simulink model "ssc_battery_management_R2020a"  (R2020a)
settings: Solver=daessc  StartTime=0.0  StopTime=2000  FixedStep=0.1  MinStep=1e-6  RelTol=1e-5  EnableMultiTasking=on
PreLoadFcn:
  | ModelPath = fileparts(get_param(bdroot,'FileName'));
  | addpath(ModelPath);
  | 
  | ssc_battery_management_R2012b_ini
values from neighbouring files (symbols this model uses):
  AltData100AMaxCurrent =     [AlternatorTableData.mat]
  AltData100AVoltage =     [AlternatorTableData.mat]
  AltData80AMaxCurrent =     [AlternatorTableData.mat]
  AltData80AVoltage =     [AlternatorTableData.mat]
  Kt = [0.80,1.10,1.20,1.12;]    [ssc_lead_acid_battery_50Ah_ini.m]    (also in ssc_lead_acid_battery_80Ah_ini.m)
  Kt_Temps = [25 40 60 75]    [ssc_lead_acid_battery_50Ah_ini.m]    (also in ssc_lead_acid_battery_80Ah_ini.m)
  theta_f = -40    [ssc_lead_acid_battery_50Ah_ini.m]    (also in ssc_lead_acid_battery_80Ah_ini.m)
  theta_init = 25    [ssc_lead_acid_battery_50Ah_ini.m]    (also in ssc_lead_acid_battery_80Ah_ini.m)
undefined symbols (not defined in the file or in its folder): beta, center, DiscIntNeverNeededParam, exponent, polyTerms, sigbuilder_block, WendlandNumTerms, width
libraries: fl_lib x130, LeadAcidBattery_lib x36, nesl_utility x28, simulink x6
(part 3 of 4)

== system ssc_battery_management_R2020a/Lead-Acid Battery/Battery Cell 5/Thermal Model ==
  Battery thermal mass : fl_lib/Thermal/Thermal Elements/Thermal Mass  mass=1 kg  sp_heat=Ctheta J/kg/K  T_specify=on  T_priority=High  T=theta_init+273 K  T_nominal_specify=off  T_nominal_unit=K  T_nominal_value=1  Q_specify=off  Q_priority=None  Q=0 W  Q_nominal_specify=off  Q_nominal_unit=W  Q_nominal_value=1
  Ideal Temperature Sensor : fl_lib/Thermal/Thermal Sensors/Temperature Sensor
  Ideal Heat Flow Source : fl_lib/Thermal/Thermal Sources/Controlled Heat Flow Rate Source
  Kt as a function of temperature : fl_lib/Physical Signals/Lookup Tables/PS Lookup Table (1D)  x=[theta_f, Kt_Temps]+273 K  f=[0 Kt]  interp_method=simscape.enum.interpolation.linear  extrap_method=simscape.enum.extrapolation.nearest
      settings: SourceProductBaseCode=SS
  Thermal Reference1 : fl_lib/Thermal/Thermal Elements/Thermal Reference
  Thermal Reference2 : fl_lib/Thermal/Thermal Elements/Thermal Reference
  Ps : PMIOPort  Tag=PMCPort  Side=Left
  H : PMIOPort  Tag=PMCPort  Port=2  Side=Left
  Kt : PMIOPort  Tag=PMCPort  Port=3  Side=Right
  T : PMIOPort  Tag=PMCPort  Port=4  Side=Right
  connections:
  Ideal Temperature Sensor/RConn1 -- Thermal Reference2/LConn1
  Ideal Temperature Sensor/RConn2 -- Kt as a function of temperature/LConn1 -- T/RConn1
  Thermal Reference1/LConn1 -- Ideal Heat Flow Source/RConn2
  H/RConn1 -- Ideal Temperature Sensor/LConn1 -- Ideal Heat Flow Source/LConn1 -- Battery thermal mass/LConn1
  Kt/RConn1 -- Kt as a function of temperature/RConn1
  Ideal Heat Flow Source/RConn1 -- Ps/RConn1

== system ssc_battery_management_R2020a/Lead-Acid Battery/Battery Cell 6/Thermal Model ==
  Battery thermal mass : fl_lib/Thermal/Thermal Elements/Thermal Mass  mass=1 kg  sp_heat=Ctheta J/kg/K  T_specify=on  T_priority=High  T=theta_init+273 K  T_nominal_specify=off  T_nominal_unit=K  T_nominal_value=1  Q_specify=off  Q_priority=None  Q=0 W  Q_nominal_specify=off  Q_nominal_unit=W  Q_nominal_value=1
  Ideal Temperature Sensor : fl_lib/Thermal/Thermal Sensors/Temperature Sensor
  Ideal Heat Flow Source : fl_lib/Thermal/Thermal Sources/Controlled Heat Flow Rate Source
  Kt as a function of temperature : fl_lib/Physical Signals/Lookup Tables/PS Lookup Table (1D)  x=[theta_f, Kt_Temps]+273 K  f=[0 Kt]  interp_method=simscape.enum.interpolation.linear  extrap_method=simscape.enum.extrapolation.nearest
      settings: SourceProductBaseCode=SS
  Thermal Reference1 : fl_lib/Thermal/Thermal Elements/Thermal Reference
  Thermal Reference2 : fl_lib/Thermal/Thermal Elements/Thermal Reference
  Ps : PMIOPort  Tag=PMCPort  Side=Left
  H : PMIOPort  Tag=PMCPort  Port=2  Side=Left
  Kt : PMIOPort  Tag=PMCPort  Port=3  Side=Right
  T : PMIOPort  Tag=PMCPort  Port=4  Side=Right
  connections:
  Ideal Temperature Sensor/RConn1 -- Thermal Reference2/LConn1
  Ideal Temperature Sensor/RConn2 -- Kt as a function of temperature/LConn1 -- T/RConn1
  Thermal Reference1/LConn1 -- Ideal Heat Flow Source/RConn2
  H/RConn1 -- Ideal Temperature Sensor/LConn1 -- Ideal Heat Flow Source/LConn1 -- Battery thermal mass/LConn1
  Kt/RConn1 -- Kt as a function of temperature/RConn1
  Ideal Heat Flow Source/RConn1 -- Ps/RConn1

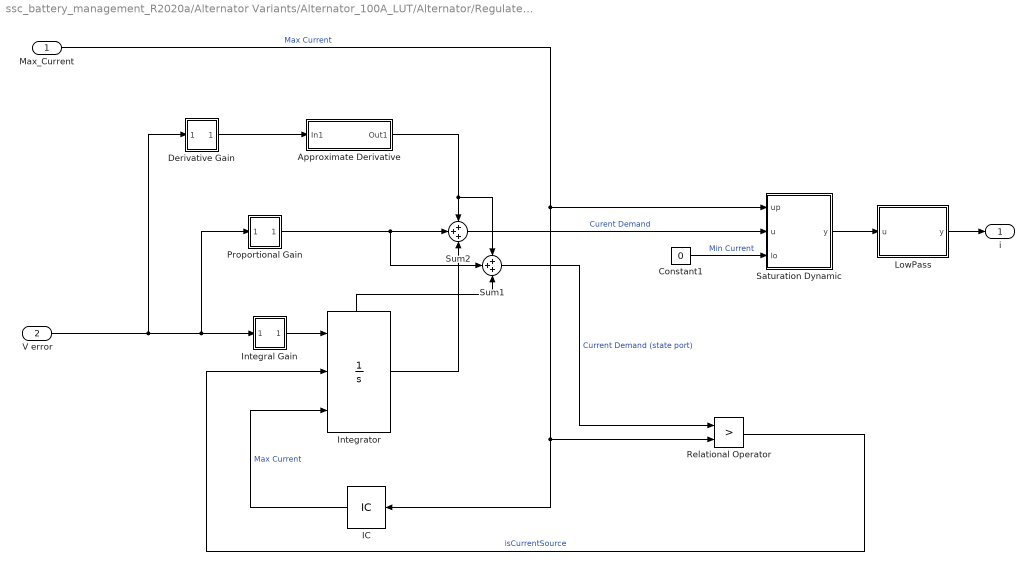
== system ssc_battery_management_R2020a/Alternator Variants/Alternator_100A_LUT/Alternator/Regulate Voltage ==
  Max_Current : Inport
  V error : Inport  Port=2
  Approximate Derivative : Subsystem
  Constant1 : Constant  Value=0  OutDataTypeStr=double
  Derivative Gain : Subsystem  LoadFcn=slideg Load  mask(Slider Gain){low=0, gain=22, high=200}
      settings: CopyFcn=slideg Copy  DeleteFcn=slideg DeleteBlock  NameChangeFcn=slideg NameChange  OpenFcn=slideg Open  CloseFcn=slideg Close  ParentCloseFcn=slideg ParentClose
      mask Display: disp(gain)
  IC : InitialCondition  Value=i_init
  Integral Gain : Subsystem  LoadFcn=slideg Load  mask(Slider Gain){low=0, gain=40, high=200}
      settings: CopyFcn=slideg Copy  DeleteFcn=slideg DeleteBlock  NameChangeFcn=slideg NameChange  OpenFcn=slideg Open  CloseFcn=slideg Close  ParentCloseFcn=slideg ParentClose
      mask Display: disp(gain)
  Integrator : Integrator  ExternalReset=falling  InitialConditionSource=external  LimitOutput=on  UpperSaturationLimit=140  LowerSaturationLimit=0  ShowStatePort=on  IgnoreLimit=on
  LowPass : Subsystem  mask{T=0.3, IC=i_init}
      mask prompts: T "Time Constant"; IC "Initial Condition"
      mask Display:
      | disp(...
      |     strvcat(['1/(' num2str(T) 's+1)'],...
      | ['IC=' num2str(IC)])...
      | )
  Proportional Gain : Subsystem  LoadFcn=slideg Load  mask(Slider Gain){low=0, gain=40, high=200}
      settings: CopyFcn=slideg Copy  DeleteFcn=slideg DeleteBlock  NameChangeFcn=slideg NameChange  OpenFcn=slideg Open  CloseFcn=slideg Close  ParentCloseFcn=slideg ParentClose
      mask Display: disp(gain)
  Relational Operator : RelationalOperator  Operator=>  OutDataTypeStr=boolean  RndMeth=Nearest
  Saturation Dynamic : Subsystem  mask(Saturation Dynamic){}
      mask help: Bound the range of the second input by using the first input (upper limit) and the third input (lower limit).
      mask Display: plot([0.15 0.85],[.5 .5],[.5 .5],[0.05 0.95],0.15+0.7*[0 .25 .75 1],0.05+0.9*[.25 .25 .75 .75]);
  Sum1 : Sum  Inputs=+++
  Sum2 : Sum  Inputs=+++
  i : Outport
  wires:
  Sum2/1 -> Saturation Dynamic/2(u)  "Curent Demand"
  Proportional Gain/1(Out1) -> Sum2/2, Sum1/2
  Integral Gain/1(Out1) -> Integrator/1
  Integrator/1 -> Sum2/3
  V error/1 -> Integral Gain/1(In1), Proportional Gain/1(In1), Derivative Gain/1(In1)
  Max_Current/1 -> Saturation Dynamic/1(up), Relational Operator/2, IC/1  "Max Current"
  Constant1/1 -> Saturation Dynamic/3(lo)  "Min Current"
  Saturation Dynamic/1(y) -> LowPass/1(u)
  Relational Operator/1 -> Integrator/2  "isCurrentSource"
  IC/1 -> Integrator/3  "Max Current"
  Approximate Derivative/1(Out1) -> Sum2/1, Sum1/1
  Derivative Gain/1(Out1) -> Approximate Derivative/1(In1)
  Integrator/State -> Sum1/3
  Sum1/1 -> Relational Operator/1  "Current Demand (state port)"
  LowPass/1(y) -> i/1

== system ssc_battery_management_R2020a/Alternator Variants/Alternator_100A_MBC/Alternator/100A_Max_Current ==
  Temp : Inport
  Voltage : Inport  Port=2
  RPM : Inport  Port=3
  Constraint Block : Subsystem
  Mx1 : Mux  Inputs=3
  xregrbf : Subsystem
      mask init:
      | xregmaskinitialization;
  Max_Current : Outport
  Constraints : Outport  Port=2
  wires:
  Constraint Block/1(C) -> Constraints/1
  xregrbf/1(Y) -> Max_Current/1
  Mx1/1 -> Constraint Block/1(X), xregrbf/1(X)
  RPM/1 -> Mx1/3
  Voltage/1 -> Mx1/2
  Temp/1 -> Mx1/1

== system ssc_battery_management_R2020a/Alternator Variants/Alternator_100A_MBC/Alternator/100A_Voltage ==
  Temp : Inport
  Load : Inport  Port=2
  RPM : Inport  Port=3
  Constraint Block : Subsystem
  Mx1 : Mux  Inputs=3
  xregrbf : Subsystem
      mask init:
      | xregmaskinitialization;
  Voltage : Outport
  Constraints : Outport  Port=2
  wires:
  Constraint Block/1(C) -> Constraints/1
  xregrbf/1(Y) -> Voltage/1
  Mx1/1 -> Constraint Block/1(X), xregrbf/1(X)
  RPM/1 -> Mx1/3
  Load/1 -> Mx1/2
  Temp/1 -> Mx1/1

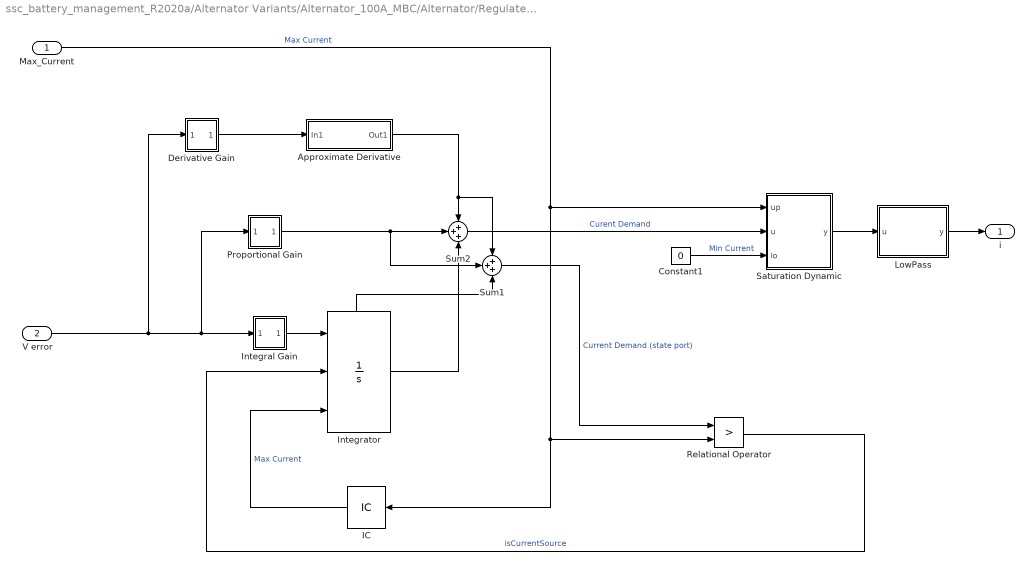
== system ssc_battery_management_R2020a/Alternator Variants/Alternator_100A_MBC/Alternator/Regulate Voltage ==
  Max_Current : Inport
  V error : Inport  Port=2
  Approximate Derivative : Subsystem
  Constant1 : Constant  Value=0  OutDataTypeStr=double
  Derivative Gain : Subsystem  LoadFcn=slideg Load  mask(Slider Gain){low=0, gain=22, high=200}
      settings: CopyFcn=slideg Copy  DeleteFcn=slideg DeleteBlock  NameChangeFcn=slideg NameChange  OpenFcn=slideg Open  CloseFcn=slideg Close  ParentCloseFcn=slideg ParentClose
      mask Display: disp(gain)
  IC : InitialCondition  Value=i_init
  Integral Gain : Subsystem  LoadFcn=slideg Load  mask(Slider Gain){low=0, gain=40, high=200}
      settings: CopyFcn=slideg Copy  DeleteFcn=slideg DeleteBlock  NameChangeFcn=slideg NameChange  OpenFcn=slideg Open  CloseFcn=slideg Close  ParentCloseFcn=slideg ParentClose
      mask Display: disp(gain)
  Integrator : Integrator  ExternalReset=falling  InitialConditionSource=external  LimitOutput=on  UpperSaturationLimit=140  LowerSaturationLimit=0  ShowStatePort=on  IgnoreLimit=on
  LowPass : Subsystem  mask{T=0.3, IC=i_init}
      mask prompts: T "Time Constant"; IC "Initial Condition"
      mask Display:
      | disp(...
      |     strvcat(['1/(' num2str(T) 's+1)'],...
      | ['IC=' num2str(IC)])...
      | )
  Proportional Gain : Subsystem  LoadFcn=slideg Load  mask(Slider Gain){low=0, gain=40, high=200}
      settings: CopyFcn=slideg Copy  DeleteFcn=slideg DeleteBlock  NameChangeFcn=slideg NameChange  OpenFcn=slideg Open  CloseFcn=slideg Close  ParentCloseFcn=slideg ParentClose
      mask Display: disp(gain)
  Relational Operator : RelationalOperator  Operator=>  OutDataTypeStr=boolean  RndMeth=Nearest
  Saturation Dynamic : Subsystem  mask(Saturation Dynamic){}
      mask help: Bound the range of the second input by using the first input (upper limit) and the third input (lower limit).
      mask Display: plot([0.15 0.85],[.5 .5],[.5 .5],[0.05 0.95],0.15+0.7*[0 .25 .75 1],0.05+0.9*[.25 .25 .75 .75]);
  Sum1 : Sum  Inputs=+++
  Sum2 : Sum  Inputs=+++
  i : Outport
  wires:
  LowPass/1(y) -> i/1
  Sum1/1 -> Relational Operator/1  "Current Demand (state port)"
  Integrator/State -> Sum1/3
  Derivative Gain/1(Out1) -> Approximate Derivative/1(In1)
  Approximate Derivative/1(Out1) -> Sum1/1, Sum2/1
  IC/1 -> Integrator/3  "Max Current"
  Relational Operator/1 -> Integrator/2  "isCurrentSource"
  Saturation Dynamic/1(y) -> LowPass/1(u)
  Constant1/1 -> Saturation Dynamic/3(lo)  "Min Current"
  Max_Current/1 -> IC/1, Relational Operator/2, Saturation Dynamic/1(up)  "Max Current"
  V error/1 -> Derivative Gain/1(In1), Proportional Gain/1(In1), Integral Gain/1(In1)
  Integrator/1 -> Sum2/3
  Integral Gain/1(Out1) -> Integrator/1
  Proportional Gain/1(Out1) -> Sum1/2, Sum2/2
  Sum2/1 -> Saturation Dynamic/2(u)  "Curent Demand"

== system ssc_battery_management_R2020a/Alternator Variants/Alternator_80A_LUT/Alternator/Regulate Voltage ==
  Max_Current : Inport
  V error : Inport  Port=2
  Approximate Derivative : Subsystem
  Constant1 : Constant  Value=0  OutDataTypeStr=double
  Derivative Gain : simulink/Math Operations/Slider Gain  gain=1  low=0  high=200
  IC : InitialCondition  Value=i_init
  Integral Gain : simulink/Math Operations/Slider Gain  gain=1  low=0  high=200
  Integrator : Integrator  ExternalReset=falling  InitialConditionSource=external  LimitOutput=on  UpperSaturationLimit=140  LowerSaturationLimit=0  ShowStatePort=on  IgnoreLimit=on
  LowPass : Subsystem  mask{T=0.3, IC=i_init}
      mask prompts: T "Time Constant"; IC "Initial Condition"
      mask Display:
      | disp(...
      |     strvcat(['1/(' num2str(T) 's+1)'],...
      | ['IC=' num2str(IC)])...
      | )
  Proportional Gain : simulink/Math Operations/Slider Gain  gain=1  low=0  high=200
  Relational Operator : RelationalOperator  Operator=>  OutDataTypeStr=boolean  RndMeth=Nearest
  Saturation Dynamic : simulink/Discontinuities/Saturation Dynamic  OutMin=[]  OutMax=[]  OutDataTypeStr=Inherit: Same as second input  OutDataType=fixdt(1, 16)  OutScaling=2^-10  DoSatur=off
  Sum1 : Sum  Inputs=+++
  Sum2 : Sum  Inputs=+++
  i : Outport
  wires:
  LowPass/1(y) -> i/1
  Sum1/1 -> Relational Operator/1  "Current Demand (state port)"
  Integrator/State -> Sum1/3
  Derivative Gain/1 -> Approximate Derivative/1(In1)
  Approximate Derivative/1(Out1) -> Sum1/1, Sum2/1
  IC/1 -> Integrator/3  "Max Current"
  Relational Operator/1 -> Integrator/2  "isCurrentSource"
  Saturation Dynamic/1 -> LowPass/1(u)
  Constant1/1 -> Saturation Dynamic/3  "Min Current"
  Max_Current/1 -> IC/1, Relational Operator/2, Saturation Dynamic/1  "Max Current"
  V error/1 -> Derivative Gain/1, Proportional Gain/1, Integral Gain/1
  Integrator/1 -> Sum2/3
  Integral Gain/1 -> Integrator/1
  Proportional Gain/1 -> Sum1/2, Sum2/2
  Sum2/1 -> Saturation Dynamic/2  "Curent Demand"

== system ssc_battery_management_R2020a/Alternator Variants/Alternator_80A_MBC/Alternator/80A_Max_Current ==
  Temp : Inport
  Voltage : Inport  Port=2
  RPM : Inport  Port=3
  Constraint Block : Subsystem
  Mx1 : Mux  Inputs=3
  xregrbf : Subsystem
      mask init:
      | xregmaskinitialization;
  Max_Current : Outport
  Constraints : Outport  Port=2
  wires:
  Constraint Block/1(C) -> Constraints/1
  xregrbf/1(Y) -> Max_Current/1
  Mx1/1 -> Constraint Block/1(X), xregrbf/1(X)
  RPM/1 -> Mx1/3
  Voltage/1 -> Mx1/2
  Temp/1 -> Mx1/1

== system ssc_battery_management_R2020a/Alternator Variants/Alternator_80A_MBC/Alternator/80A_Voltage ==
  Temp : Inport
  Load : Inport  Port=2
  RPM : Inport  Port=3
  Constraint Block : Subsystem
  Mx1 : Mux  Inputs=3
  xregrbf : Subsystem
      mask init:
      | xregmaskinitialization;
  Voltage : Outport
  Constraints : Outport  Port=2
  wires:
  Constraint Block/1(C) -> Constraints/1
  xregrbf/1(Y) -> Voltage/1
  Mx1/1 -> Constraint Block/1(X), xregrbf/1(X)
  RPM/1 -> Mx1/3
  Load/1 -> Mx1/2
  Temp/1 -> Mx1/1

== system ssc_battery_management_R2020a/Alternator Variants/Alternator_80A_MBC/Alternator/Regulate Voltage ==
  Max_Current : Inport
  V error : Inport  Port=2
  Approximate Derivative : Subsystem
  Constant1 : Constant  Value=0  OutDataTypeStr=double
  Derivative Gain : Subsystem  LoadFcn=slideg Load  mask(Slider Gain){low=0, gain=22, high=200}
      settings: CopyFcn=slideg Copy  DeleteFcn=slideg DeleteBlock  NameChangeFcn=slideg NameChange  OpenFcn=slideg Open  CloseFcn=slideg Close  ParentCloseFcn=slideg ParentClose
      mask Display: disp(gain)
  IC : InitialCondition  Value=i_init
  Integral Gain : Subsystem  LoadFcn=slideg Load  mask(Slider Gain){low=0, gain=40, high=200}
      settings: CopyFcn=slideg Copy  DeleteFcn=slideg DeleteBlock  NameChangeFcn=slideg NameChange  OpenFcn=slideg Open  CloseFcn=slideg Close  ParentCloseFcn=slideg ParentClose
      mask Display: disp(gain)
  Integrator : Integrator  ExternalReset=falling  InitialConditionSource=external  LimitOutput=on  UpperSaturationLimit=140  LowerSaturationLimit=0  ShowStatePort=on  IgnoreLimit=on
  LowPass : Subsystem  mask{T=0.3, IC=i_init}
      mask prompts: T "Time Constant"; IC "Initial Condition"
      mask Display:
      | disp(...
      |     strvcat(['1/(' num2str(T) 's+1)'],...
      | ['IC=' num2str(IC)])...
      | )
  Proportional Gain : Subsystem  LoadFcn=slideg Load  mask(Slider Gain){low=0, gain=40, high=200}
      settings: CopyFcn=slideg Copy  DeleteFcn=slideg DeleteBlock  NameChangeFcn=slideg NameChange  OpenFcn=slideg Open  CloseFcn=slideg Close  ParentCloseFcn=slideg ParentClose
      mask Display: disp(gain)
  Relational Operator : RelationalOperator  Operator=>  OutDataTypeStr=boolean  RndMeth=Nearest
  Saturation Dynamic : Subsystem  mask(Saturation Dynamic){}
      mask help: Bound the range of the second input by using the first input (upper limit) and the third input (lower limit).
      mask Display: plot([0.15 0.85],[.5 .5],[.5 .5],[0.05 0.95],0.15+0.7*[0 .25 .75 1],0.05+0.9*[.25 .25 .75 .75]);
  Sum1 : Sum  Inputs=+++
  Sum2 : Sum  Inputs=+++
  i : Outport
  wires:
  Sum2/1 -> Saturation Dynamic/2(u)  "Curent Demand"
  Proportional Gain/1(Out1) -> Sum2/2, Sum1/2
  Integral Gain/1(Out1) -> Integrator/1
  Integrator/1 -> Sum2/3
  V error/1 -> Integral Gain/1(In1), Proportional Gain/1(In1), Derivative Gain/1(In1)
  Max_Current/1 -> Saturation Dynamic/1(up), Relational Operator/2, IC/1  "Max Current"
  Constant1/1 -> Saturation Dynamic/3(lo)  "Min Current"
  Saturation Dynamic/1(y) -> LowPass/1(u)
  Relational Operator/1 -> Integrator/2  "isCurrentSource"
  IC/1 -> Integrator/3  "Max Current"
  Approximate Derivative/1(Out1) -> Sum2/1, Sum1/1
  Derivative Gain/1(Out1) -> Approximate Derivative/1(In1)
  Integrator/State -> Sum1/3
  Sum1/1 -> Relational Operator/1  "Current Demand (state port)"
  LowPass/1(y) -> i/1

== system ssc_battery_management_R2020a/Alternator Variants/Alternator_100A_LUT/Alternator/Regulate Voltage/Approximate Derivative ==
  In1 : Inport
  Derivative Gain : Subsystem  LoadFcn=slideg Load  mask(Slider Gain){low=0, gain=38, high=200}
      settings: CopyFcn=slideg Copy  DeleteFcn=slideg DeleteBlock  NameChangeFcn=slideg NameChange  OpenFcn=slideg Open  CloseFcn=slideg Close  ParentCloseFcn=slideg ParentClose
      mask Display: disp(gain)
  Filter : Integrator
  Sum3 : Sum  Inputs=|+-  InputSameDT=on  SaturateOnIntegerOverflow=on  OutDataTypeStr=Inherit: Same as first input
  Out1 : Outport
  wires:
  In1/1 -> Sum3/1
  Filter/1 -> Sum3/2
  Derivative Gain/1(Out1) -> Out1/1, Filter/1
  Sum3/1 -> Derivative Gain/1(In1)

== system ssc_battery_management_R2020a/Alternator Variants/Alternator_100A_LUT/Alternator/Regulate Voltage/Derivative Gain ==
  In1 : Inport
  Slider Gain : Gain  Gain=gain  SaturateOnIntegerOverflow=on  OutDataTypeStr=Inherit: Same as input  ParamDataTypeStr=Inherit: Same as input
  Out1 : Outport
  wires:
  In1/1 -> Slider Gain/1
  Slider Gain/1 -> Out1/1

== system ssc_battery_management_R2020a/Alternator Variants/Alternator_100A_LUT/Alternator/Regulate Voltage/Integral Gain ==
  In1 : Inport
  Slider Gain : Gain  Gain=gain  SaturateOnIntegerOverflow=on  OutDataTypeStr=Inherit: Same as input  ParamDataTypeStr=Inherit: Same as input
  Out1 : Outport
  wires:
  Slider Gain/1 -> Out1/1
  In1/1 -> Slider Gain/1

== system ssc_battery_management_R2020a/Alternator Variants/Alternator_100A_LUT/Alternator/Regulate Voltage/LowPass ==
  u : Inport
  Gain : Gain  Gain=1/T
  Integrator : Integrator  InitialCondition=IC
  Sum : Sum  Inputs=|+-
  y : Outport
  wires:
  Gain/1 -> Integrator/1  "ydot"
  u/1 -> Sum/1
  Sum/1 -> Gain/1  "ydot"
  Integrator/1 -> y/1, Sum/2  "y"

== system ssc_battery_management_R2020a/Alternator Variants/Alternator_100A_LUT/Alternator/Regulate Voltage/Proportional Gain ==
  In1 : Inport
  Slider Gain : Gain  Gain=gain  SaturateOnIntegerOverflow=on  OutDataTypeStr=Inherit: Same as input  ParamDataTypeStr=Inherit: Same as input
  Out1 : Outport
  wires:
  Slider Gain/1 -> Out1/1
  In1/1 -> Slider Gain/1

== system ssc_battery_management_R2020a/Alternator Variants/Alternator_100A_LUT/Alternator/Regulate Voltage/Saturation Dynamic ==
  up : Inport
  u : Inport  Port=2
  lo : Inport  Port=3
  Enforce lower limit : MinMax  Function=max  Inputs=2  OutDataTypeStr=Inherit: Inherit via back propagation  ZeroCross=off
  Enforce upper limit : MinMax  Inputs=2  OutDataTypeStr=Inherit: Inherit via back propagation  ZeroCross=off
  FixPt Data Type Duplicate : S-Function  FunctionName=sfix_dtprop  Parameters=15,NumInputPorts  SFunctionDeploymentMode=off  EnableBusSupport=off  mask(Data Type Duplicate){NumInputPorts=3}
      mask prompts: NumInputPorts "Number of input ports:"
      mask help: Force all inputs to have the exact same data type.
      mask Display: fprintf('Same\nDT')
  y : Outport
  wires:
  lo/1 -> Enforce lower limit/1
  Enforce lower limit/1 -> FixPt Data Type Duplicate/2, Enforce upper limit/1
  u/1 -> Enforce lower limit/2, FixPt Data Type Duplicate/3
  up/1 -> Enforce upper limit/2
  Enforce upper limit/1 -> y/1, FixPt Data Type Duplicate/1

== system ssc_battery_management_R2020a/Alternator Variants/Alternator_100A_MBC/Alternator/100A_Max_Current/Constraint Block ==
  X : Inport
  Constraints : Subsystem
  Term : Terminator
  C : Outport
  wires:
  Constraints/2(Distances) -> C/1
  Constraints/1(Status) -> Term/1
  X/1 -> Constraints/1(Factors)

== system ssc_battery_management_R2020a/Alternator Variants/Alternator_100A_MBC/Alternator/100A_Max_Current/xregrbf ==
  X : Inport
  Code : Subsystem
  Saturation : Saturate  UpperLimit=1  LowerLimit=-1  ZeroCross=off
  rbfwendlandEval : Subsystem  mask{NumTerms=WendlandNumTerms, E=exponent, P=polyTerms, B=beta, S=width, C=center}
      mask prompts: NumTerms "Number of Poylnomial Terms"; E "Exponent"; P "Polynomial Terms"; B "Betas"; S "Widths"; C "Centers"
  term : Terminator
  Y : Outport
  wires:
  Saturation/1 -> rbfwendlandEval/1(X)
  rbfwendlandEval/2(J) -> term/1
  rbfwendlandEval/1(Y) -> Y/1
  Code/1(XCoded) -> Saturation/1
  X/1 -> Code/1(XIn)

== system ssc_battery_management_R2020a/Alternator Variants/Alternator_100A_MBC/Alternator/100A_Voltage/Constraint Block ==
  X : Inport
  Constraints : Subsystem
  Term : Terminator
  C : Outport
  wires:
  Constraints/2(Distances) -> C/1
  Constraints/1(Status) -> Term/1
  X/1 -> Constraints/1(Factors)

== system ssc_battery_management_R2020a/Alternator Variants/Alternator_100A_MBC/Alternator/100A_Voltage/xregrbf ==
  X : Inport
  Code : Subsystem
  Saturation : Saturate  UpperLimit=1  LowerLimit=-1  ZeroCross=off
  rbfwendlandEval : Subsystem  mask{NumTerms=WendlandNumTerms, E=exponent, P=polyTerms, B=beta, S=width, C=center}
      mask prompts: NumTerms "Number of Poylnomial Terms"; E "Exponent"; P "Polynomial Terms"; B "Betas"; S "Widths"; C "Centers"
  term : Terminator
  Y : Outport
  wires:
  Saturation/1 -> rbfwendlandEval/1(X)
  rbfwendlandEval/2(J) -> term/1
  rbfwendlandEval/1(Y) -> Y/1
  Code/1(XCoded) -> Saturation/1
  X/1 -> Code/1(XIn)

== system ssc_battery_management_R2020a/Alternator Variants/Alternator_100A_MBC/Alternator/Regulate Voltage/Approximate Derivative ==
  In1 : Inport
  Derivative Gain : Subsystem  LoadFcn=slideg Load  mask(Slider Gain){low=0, gain=38, high=200}
      settings: CopyFcn=slideg Copy  DeleteFcn=slideg DeleteBlock  NameChangeFcn=slideg NameChange  OpenFcn=slideg Open  CloseFcn=slideg Close  ParentCloseFcn=slideg ParentClose
      mask Display: disp(gain)
  Filter : Integrator
  Sum3 : Sum  Inputs=|+-  InputSameDT=on  SaturateOnIntegerOverflow=on  OutDataTypeStr=Inherit: Same as first input
  Out1 : Outport
  wires:
  Sum3/1 -> Derivative Gain/1(In1)
  Derivative Gain/1(Out1) -> Filter/1, Out1/1
  Filter/1 -> Sum3/2
  In1/1 -> Sum3/1

== system ssc_battery_management_R2020a/Alternator Variants/Alternator_100A_MBC/Alternator/Regulate Voltage/Derivative Gain ==
  In1 : Inport
  Slider Gain : Gain  Gain=gain  SaturateOnIntegerOverflow=on  OutDataTypeStr=Inherit: Same as input  ParamDataTypeStr=Inherit: Same as input
  Out1 : Outport
  wires:
  Slider Gain/1 -> Out1/1
  In1/1 -> Slider Gain/1

== system ssc_battery_management_R2020a/Alternator Variants/Alternator_100A_MBC/Alternator/Regulate Voltage/Integral Gain ==
  In1 : Inport
  Slider Gain : Gain  Gain=gain  SaturateOnIntegerOverflow=on  OutDataTypeStr=Inherit: Same as input  ParamDataTypeStr=Inherit: Same as input
  Out1 : Outport
  wires:
  In1/1 -> Slider Gain/1
  Slider Gain/1 -> Out1/1

== system ssc_battery_management_R2020a/Alternator Variants/Alternator_100A_MBC/Alternator/Regulate Voltage/LowPass ==
  u : Inport
  Gain : Gain  Gain=1/T
  Integrator : Integrator  InitialCondition=IC
  Sum : Sum  Inputs=|+-
  y : Outport
  wires:
  Integrator/1 -> Sum/2, y/1  "y"
  Sum/1 -> Gain/1  "ydot"
  u/1 -> Sum/1
  Gain/1 -> Integrator/1  "ydot"

== system ssc_battery_management_R2020a/Alternator Variants/Alternator_100A_MBC/Alternator/Regulate Voltage/Proportional Gain ==
  In1 : Inport
  Slider Gain : Gain  Gain=gain  SaturateOnIntegerOverflow=on  OutDataTypeStr=Inherit: Same as input  ParamDataTypeStr=Inherit: Same as input
  Out1 : Outport
  wires:
  In1/1 -> Slider Gain/1
  Slider Gain/1 -> Out1/1

== system ssc_battery_management_R2020a/Alternator Variants/Alternator_100A_MBC/Alternator/Regulate Voltage/Saturation Dynamic ==
  up : Inport
  u : Inport  Port=2
  lo : Inport  Port=3
  Enforce lower limit : MinMax  Function=max  Inputs=2  OutDataTypeStr=Inherit: Inherit via back propagation  ZeroCross=off
  Enforce upper limit : MinMax  Inputs=2  OutDataTypeStr=Inherit: Inherit via back propagation  ZeroCross=off
  FixPt Data Type Duplicate : S-Function  FunctionName=sfix_dtprop  Parameters=15,NumInputPorts  SFunctionDeploymentMode=off  EnableBusSupport=off  mask(Data Type Duplicate){NumInputPorts=3}
      mask prompts: NumInputPorts "Number of input ports:"
      mask help: Force all inputs to have the exact same data type.
      mask Display: fprintf('Same\nDT')
  y : Outport
  wires:
  Enforce upper limit/1 -> FixPt Data Type Duplicate/1, y/1
  up/1 -> Enforce upper limit/2
  u/1 -> FixPt Data Type Duplicate/3, Enforce lower limit/2
  Enforce lower limit/1 -> Enforce upper limit/1, FixPt Data Type Duplicate/2
  lo/1 -> Enforce lower limit/1

== system ssc_battery_management_R2020a/Alternator Variants/Alternator_80A_LUT/Alternator/Regulate Voltage/Approximate Derivative ==
  In1 : Inport
  Derivative Gain : simulink/Math Operations/Slider Gain  gain=1  low=0  high=200
  Filter : Integrator
  Sum3 : Sum  Inputs=|+-  InputSameDT=on  SaturateOnIntegerOverflow=on  OutDataTypeStr=Inherit: Same as first input
  Out1 : Outport
  wires:
  Sum3/1 -> Derivative Gain/1
  Derivative Gain/1 -> Filter/1, Out1/1
  Filter/1 -> Sum3/2
  In1/1 -> Sum3/1

== system ssc_battery_management_R2020a/Alternator Variants/Alternator_80A_LUT/Alternator/Regulate Voltage/LowPass ==
  u : Inport
  Gain : Gain  Gain=1/T
  Integrator : Integrator  InitialCondition=IC
  Sum : Sum  Inputs=|+-
  y : Outport
  wires:
  Integrator/1 -> Sum/2, y/1  "y"
  Sum/1 -> Gain/1  "ydot"
  u/1 -> Sum/1
  Gain/1 -> Integrator/1  "ydot"

== system ssc_battery_management_R2020a/Alternator Variants/Alternator_80A_MBC/Alternator/80A_Max_Current/Constraint Block ==
  X : Inport
  Constraints : Subsystem
  Term : Terminator
  C : Outport
  wires:
  Constraints/2(Distances) -> C/1
  Constraints/1(Status) -> Term/1
  X/1 -> Constraints/1(Factors)

== system ssc_battery_management_R2020a/Alternator Variants/Alternator_80A_MBC/Alternator/80A_Max_Current/xregrbf ==
  X : Inport
  Code : Subsystem
  Saturation : Saturate  UpperLimit=1  LowerLimit=-1  ZeroCross=off
  rbflogisticrbfEval : Subsystem  mask{B=beta, S=width, C=center}
      mask prompts: B "Betas"; S "Widths"; C "Centers"
  term : Terminator
  Y : Outport
  wires:
  Saturation/1 -> rbflogisticrbfEval/1(X)
  rbflogisticrbfEval/2(J) -> term/1
  rbflogisticrbfEval/1(Y) -> Y/1
  Code/1(XCoded) -> Saturation/1
  X/1 -> Code/1(XIn)

== system ssc_battery_management_R2020a/Alternator Variants/Alternator_80A_MBC/Alternator/80A_Voltage/Constraint Block ==
  X : Inport
  Constraints : Subsystem
  Term : Terminator
  C : Outport
  wires:
  Constraints/2(Distances) -> C/1
  Constraints/1(Status) -> Term/1
  X/1 -> Constraints/1(Factors)

== system ssc_battery_management_R2020a/Alternator Variants/Alternator_80A_MBC/Alternator/80A_Voltage/xregrbf ==
  X : Inport
  Code : Subsystem
  Saturation : Saturate  UpperLimit=1  LowerLimit=-1  ZeroCross=off
  rbfwendlandEval : Subsystem  mask{NumTerms=WendlandNumTerms, E=exponent, P=polyTerms, B=beta, S=width, C=center}
      mask prompts: NumTerms "Number of Poylnomial Terms"; E "Exponent"; P "Polynomial Terms"; B "Betas"; S "Widths"; C "Centers"
  term : Terminator
  Y : Outport
  wires:
  Saturation/1 -> rbfwendlandEval/1(X)
  rbfwendlandEval/2(J) -> term/1
  rbfwendlandEval/1(Y) -> Y/1
  Code/1(XCoded) -> Saturation/1
  X/1 -> Code/1(XIn)

== system ssc_battery_management_R2020a/Alternator Variants/Alternator_80A_MBC/Alternator/Regulate Voltage/Approximate Derivative ==
  In1 : Inport
  Derivative Gain : Subsystem  LoadFcn=slideg Load  mask(Slider Gain){low=0, gain=38, high=200}
      settings: CopyFcn=slideg Copy  DeleteFcn=slideg DeleteBlock  NameChangeFcn=slideg NameChange  OpenFcn=slideg Open  CloseFcn=slideg Close  ParentCloseFcn=slideg ParentClose
      mask Display: disp(gain)
  Filter : Integrator
  Sum3 : Sum  Inputs=|+-  InputSameDT=on  SaturateOnIntegerOverflow=on  OutDataTypeStr=Inherit: Same as first input
  Out1 : Outport
  wires:
  In1/1 -> Sum3/1
  Filter/1 -> Sum3/2
  Derivative Gain/1(Out1) -> Out1/1, Filter/1
  Sum3/1 -> Derivative Gain/1(In1)

== system ssc_battery_management_R2020a/Alternator Variants/Alternator_80A_MBC/Alternator/Regulate Voltage/Derivative Gain ==
  In1 : Inport
  Slider Gain : Gain  Gain=gain  SaturateOnIntegerOverflow=on  OutDataTypeStr=Inherit: Same as input  ParamDataTypeStr=Inherit: Same as input
  Out1 : Outport
  wires:
  In1/1 -> Slider Gain/1
  Slider Gain/1 -> Out1/1

== system ssc_battery_management_R2020a/Alternator Variants/Alternator_80A_MBC/Alternator/Regulate Voltage/Integral Gain ==
  In1 : Inport
  Slider Gain : Gain  Gain=gain  SaturateOnIntegerOverflow=on  OutDataTypeStr=Inherit: Same as input  ParamDataTypeStr=Inherit: Same as input
  Out1 : Outport
  wires:
  Slider Gain/1 -> Out1/1
  In1/1 -> Slider Gain/1

== system ssc_battery_management_R2020a/Alternator Variants/Alternator_80A_MBC/Alternator/Regulate Voltage/LowPass ==
  u : Inport
  Gain : Gain  Gain=1/T
  Integrator : Integrator  InitialCondition=IC
  Sum : Sum  Inputs=|+-
  y : Outport
  wires:
  Gain/1 -> Integrator/1  "ydot"
  u/1 -> Sum/1
  Sum/1 -> Gain/1  "ydot"
  Integrator/1 -> y/1, Sum/2  "y"

== system ssc_battery_management_R2020a/Alternator Variants/Alternator_80A_MBC/Alternator/Regulate Voltage/Proportional Gain ==
  In1 : Inport
  Slider Gain : Gain  Gain=gain  SaturateOnIntegerOverflow=on  OutDataTypeStr=Inherit: Same as input  ParamDataTypeStr=Inherit: Same as input
  Out1 : Outport
  wires:
  Slider Gain/1 -> Out1/1
  In1/1 -> Slider Gain/1

== system ssc_battery_management_R2020a/Alternator Variants/Alternator_80A_MBC/Alternator/Regulate Voltage/Saturation Dynamic ==
  up : Inport
  u : Inport  Port=2
  lo : Inport  Port=3
  Enforce lower limit : MinMax  Function=max  Inputs=2  OutDataTypeStr=Inherit: Inherit via back propagation  ZeroCross=off
  Enforce upper limit : MinMax  Inputs=2  OutDataTypeStr=Inherit: Inherit via back propagation  ZeroCross=off
  FixPt Data Type Duplicate : S-Function  FunctionName=sfix_dtprop  Parameters=15,NumInputPorts  SFunctionDeploymentMode=off  EnableBusSupport=off  mask(Data Type Duplicate){NumInputPorts=3}
      mask prompts: NumInputPorts "Number of input ports:"
      mask help: Force all inputs to have the exact same data type.
      mask Display: fprintf('Same\nDT')
  y : Outport
  wires:
  lo/1 -> Enforce lower limit/1
  Enforce lower limit/1 -> FixPt Data Type Duplicate/2, Enforce upper limit/1
  u/1 -> Enforce lower limit/2, FixPt Data Type Duplicate/3
  up/1 -> Enforce upper limit/2
  Enforce upper limit/1 -> y/1, FixPt Data Type Duplicate/1

== system ssc_battery_management_R2020a/Alternator Variants/Alternator_100A_LUT/Alternator/Regulate Voltage/Approximate Derivative/Derivative Gain ==
  In1 : Inport
  Slider Gain : Gain  Gain=gain  SaturateOnIntegerOverflow=on  OutDataTypeStr=Inherit: Same as input  ParamDataTypeStr=Inherit: Same as input
  Out1 : Outport
  wires:
  In1/1 -> Slider Gain/1
  Slider Gain/1 -> Out1/1

== system ssc_battery_management_R2020a/Alternator Variants/Alternator_100A_MBC/Alternator/100A_Max_Current/Constraint Block/Constraints ==
  Factors : Inport
  Compare : RelationalOperator  Operator=<=  RndMeth=Nearest  InputSameDT=on
  Constant : Constant  Value=0
  Constraint : Subsystem  mask(MBC Constraint){}
      mask help: This is a constraint generated by the Model-Based Calibration Toolbox.
      mask Display:
      | disp( 'MBC\nConstraint' )
      | port_label( 'output', 1, 'In/Out' )
  T : Terminator
  Status : Outport
  Distances : Outport  Port=2
  wires:
  Constraint/2(Interior Point) -> T/1
  Constraint/1(Distance) -> Compare/1, Distances/1
  Factors/1 -> Constraint/1(Xin)
  Compare/1 -> Status/1
  Constant/1 -> Compare/2

== system ssc_battery_management_R2020a/Alternator Variants/Alternator_100A_MBC/Alternator/100A_Max_Current/xregrbf/Code ==
  XIn : Inport
  Mid : Constant  Value=[45 12.75 3500 ]
  demux : Demux  Outputs=3
      settings: DisplayOption=none
  gain : Gain  Gain=[0.0153846153846154 0.8 0.0004 ]  SaturateOnIntegerOverflow=on  OutDataTypeStr=Inherit: Same as input  ParamDataTypeStr=Inherit: Same as input
  mux : Mux  Inputs=3
  sum : Sum  Inputs=-+|  InputSameDT=on  SaturateOnIntegerOverflow=on  OutDataTypeStr=Inherit: Same as first input
  XCoded : Outport
  wires:
  gain/1 -> XCoded/1
  sum/1 -> gain/1
  mux/1 -> sum/2
  XIn/1 -> demux/1
  Mid/1 -> sum/1
  demux/3 -> mux/3
  demux/2 -> mux/2
  demux/1 -> mux/1

== system ssc_battery_management_R2020a/Alternator Variants/Alternator_100A_MBC/Alternator/100A_Max_Current/xregrbf/rbfwendlandEval ==
  X : Inport
  Constant13 : Constant  Value=P
  Constant14 : Constant  Value=E
  Constant2 : Constant  Value=S  VectorParams1D=off
  Constant3 : Constant  Value=B
  Constant4 : Constant  Value=C  VectorParams1D=off
  Math Function4 : Math  Operator=sqrt  SignedPower=on  SaturateOnIntegerOverflow=on
  Product4 : Product  Multiplication=Matrix(*)  InputSameDT=on  SaturateOnIntegerOverflow=on  OutDataTypeStr=Inherit: Same as first input
  R : Subsystem
  Wendland : Subsystem  mask{NumTerms=NumTerms}
      mask prompts: NumTerms "Number of Polynomial Terms"
  Y : Outport
  J : Outport  Port=2
  wires:
  Constant14/1 -> Wendland/3(Exponent)
  Product4/1 -> Y/1
  Wendland/1(P) -> J/1, Product4/1
  Constant3/1 -> Product4/2
  Math Function4/1 -> Wendland/1(R/S)
  Constant4/1 -> R/2("Centers ")
  X/1 -> R/1(X)
  Constant2/1 -> R/3(S)
  R/1((R/S)^2) -> Math Function4/1
  Constant13/1 -> Wendland/2(PolyTerms)

== system ssc_battery_management_R2020a/Alternator Variants/Alternator_100A_MBC/Alternator/100A_Voltage/Constraint Block/Constraints ==
  Factors : Inport
  Compare : RelationalOperator  Operator=<=  RndMeth=Nearest  InputSameDT=on
  Constant : Constant  Value=0
  Constraint : Subsystem  mask(MBC Constraint){}
      mask help: This is a constraint generated by the Model-Based Calibration Toolbox.
      mask Display:
      | disp( 'MBC\nConstraint' )
      | port_label( 'output', 1, 'In/Out' )
  T : Terminator
  Status : Outport
  Distances : Outport  Port=2
  wires:
  Constraint/2(Interior Point) -> T/1
  Constraint/1(Distance) -> Compare/1, Distances/1
  Factors/1 -> Constraint/1(Xin)
  Compare/1 -> Status/1
  Constant/1 -> Compare/2

== system ssc_battery_management_R2020a/Alternator Variants/Alternator_100A_MBC/Alternator/100A_Voltage/xregrbf/Code ==
  XIn : Inport
  Mid : Constant  Value=[45 70 3500 ]
  demux : Demux  Outputs=3
      settings: DisplayOption=none
  gain : Gain  Gain=[0.0153846153846154 0.02 0.0004 ]  SaturateOnIntegerOverflow=on  OutDataTypeStr=Inherit: Same as input  ParamDataTypeStr=Inherit: Same as input
  mux : Mux  Inputs=3
  sum : Sum  Inputs=-+|  InputSameDT=on  SaturateOnIntegerOverflow=on  OutDataTypeStr=Inherit: Same as first input
  XCoded : Outport
  wires:
  gain/1 -> XCoded/1
  sum/1 -> gain/1
  mux/1 -> sum/2
  XIn/1 -> demux/1
  Mid/1 -> sum/1
  demux/3 -> mux/3
  demux/2 -> mux/2
  demux/1 -> mux/1

== system ssc_battery_management_R2020a/Alternator Variants/Alternator_100A_MBC/Alternator/100A_Voltage/xregrbf/rbfwendlandEval ==
  X : Inport
  Constant13 : Constant  Value=P
  Constant14 : Constant  Value=E
  Constant2 : Constant  Value=S  VectorParams1D=off
  Constant3 : Constant  Value=B
  Constant4 : Constant  Value=C  VectorParams1D=off
  Math Function4 : Math  Operator=sqrt  SignedPower=on  SaturateOnIntegerOverflow=on
  Product4 : Product  Multiplication=Matrix(*)  InputSameDT=on  SaturateOnIntegerOverflow=on  OutDataTypeStr=Inherit: Same as first input
  R : Subsystem
  Wendland : Subsystem  mask{NumTerms=NumTerms}
      mask prompts: NumTerms "Number of Polynomial Terms"
  Y : Outport
  J : Outport  Port=2
  wires:
  Constant14/1 -> Wendland/3(Exponent)
  Product4/1 -> Y/1
  Wendland/1(P) -> J/1, Product4/1
  Constant3/1 -> Product4/2
  Math Function4/1 -> Wendland/1(R/S)
  Constant4/1 -> R/2("Centers ")
  X/1 -> R/1(X)
  Constant2/1 -> R/3(S)
  R/1((R/S)^2) -> Math Function4/1
  Constant13/1 -> Wendland/2(PolyTerms)

== system ssc_battery_management_R2020a/Alternator Variants/Alternator_100A_MBC/Alternator/Regulate Voltage/Approximate Derivative/Derivative Gain ==
  In1 : Inport
  Slider Gain : Gain  Gain=gain  SaturateOnIntegerOverflow=on  OutDataTypeStr=Inherit: Same as input  ParamDataTypeStr=Inherit: Same as input
  Out1 : Outport
  wires:
  Slider Gain/1 -> Out1/1
  In1/1 -> Slider Gain/1

== system ssc_battery_management_R2020a/Alternator Variants/Alternator_80A_MBC/Alternator/80A_Max_Current/Constraint Block/Constraints ==
  Factors : Inport
  Compare : RelationalOperator  Operator=<=  RndMeth=Nearest  InputSameDT=on
  Constant : Constant  Value=0
  Constraint : Subsystem  mask(MBC Constraint){}
      mask help: This is a constraint generated by the Model-Based Calibration Toolbox.
      mask Display:
      | disp( 'MBC\nConstraint' )
      | port_label( 'output', 1, 'In/Out' )
  T : Terminator
  Status : Outport
  Distances : Outport  Port=2
  wires:
  Constraint/2(Interior Point) -> T/1
  Constraint/1(Distance) -> Compare/1, Distances/1
  Factors/1 -> Constraint/1(Xin)
  Compare/1 -> Status/1
  Constant/1 -> Compare/2

== system ssc_battery_management_R2020a/Alternator Variants/Alternator_80A_MBC/Alternator/80A_Max_Current/xregrbf/Code ==
  XIn : Inport
  Mid : Constant  Value=[35 12.75 3500 ]
  demux : Demux  Outputs=3
      settings: DisplayOption=none
  gain : Gain  Gain=[0.0181818181818182 0.8 0.0004 ]  SaturateOnIntegerOverflow=on  OutDataTypeStr=Inherit: Same as input  ParamDataTypeStr=Inherit: Same as input
  mux : Mux  Inputs=3
  sum : Sum  Inputs=-+|  InputSameDT=on  SaturateOnIntegerOverflow=on  OutDataTypeStr=Inherit: Same as first input
  XCoded : Outport
  wires:
  gain/1 -> XCoded/1
  sum/1 -> gain/1
  mux/1 -> sum/2
  XIn/1 -> demux/1
  Mid/1 -> sum/1
  demux/3 -> mux/3
  demux/2 -> mux/2
  demux/1 -> mux/1

== system ssc_battery_management_R2020a/Alternator Variants/Alternator_80A_MBC/Alternator/80A_Max_Current/xregrbf/rbflogisticrbfEval ==
  X : Inport
  Constant2 : Constant  Value=S  VectorParams1D=off
  Constant3 : Constant  Value=B
  Constant4 : Constant  Value=C  VectorParams1D=off
  Logistic : Subsystem
  Math Function4 : Math  Operator=sqrt  SignedPower=on  SaturateOnIntegerOverflow=on
  Product4 : Product  Multiplication=Matrix(*)  InputSameDT=on  SaturateOnIntegerOverflow=on  OutDataTypeStr=Inherit: Same as first input
  R : Subsystem
  Y : Outport
  J : Outport  Port=2
  wires:
  Math Function4/1 -> Logistic/1(R/S)
  Constant3/1 -> Product4/2
  R/1((R/S)^2) -> Math Function4/1
  Logistic/1(P) -> J/1, Product4/1
  Product4/1 -> Y/1
  Constant4/1 -> R/2("Centers ")
  X/1 -> R/1(X)
  Constant2/1 -> R/3(S)

== system ssc_battery_management_R2020a/Alternator Variants/Alternator_80A_MBC/Alternator/80A_Voltage/Constraint Block/Constraints ==
  Factors : Inport
  Compare : RelationalOperator  Operator=<=  RndMeth=Nearest  InputSameDT=on
  Constant : Constant  Value=0
  Constraint : Subsystem  mask(MBC Constraint){}
      mask help: This is a constraint generated by the Model-Based Calibration Toolbox.
      mask Display:
      | disp( 'MBC\nConstraint' )
      | port_label( 'output', 1, 'In/Out' )
  T : Terminator
  Status : Outport
  Distances : Outport  Port=2
  wires:
  Constraint/2(Interior Point) -> T/1
  Constraint/1(Distance) -> Compare/1, Distances/1
  Factors/1 -> Constraint/1(Xin)
  Compare/1 -> Status/1
  Constant/1 -> Compare/2

== system ssc_battery_management_R2020a/Alternator Variants/Alternator_80A_MBC/Alternator/80A_Voltage/xregrbf/Code ==
  XIn : Inport
  Mid : Constant  Value=[45 70 3500 ]
  demux : Demux  Outputs=3
      settings: DisplayOption=none
  gain : Gain  Gain=[0.0153846153846154 0.02 0.0004 ]  SaturateOnIntegerOverflow=on  OutDataTypeStr=Inherit: Same as input  ParamDataTypeStr=Inherit: Same as input
  mux : Mux  Inputs=3
  sum : Sum  Inputs=-+|  InputSameDT=on  SaturateOnIntegerOverflow=on  OutDataTypeStr=Inherit: Same as first input
  XCoded : Outport
  wires:
  gain/1 -> XCoded/1
  sum/1 -> gain/1
  mux/1 -> sum/2
  XIn/1 -> demux/1
  Mid/1 -> sum/1
  demux/3 -> mux/3
  demux/2 -> mux/2
  demux/1 -> mux/1

== system ssc_battery_management_R2020a/Alternator Variants/Alternator_80A_MBC/Alternator/80A_Voltage/xregrbf/rbfwendlandEval ==
  X : Inport
  Constant13 : Constant  Value=P
  Constant14 : Constant  Value=E
  Constant2 : Constant  Value=S  VectorParams1D=off
  Constant3 : Constant  Value=B
  Constant4 : Constant  Value=C  VectorParams1D=off
  Math Function4 : Math  Operator=sqrt  SignedPower=on  SaturateOnIntegerOverflow=on
  Product4 : Product  Multiplication=Matrix(*)  InputSameDT=on  SaturateOnIntegerOverflow=on  OutDataTypeStr=Inherit: Same as first input
  R : Subsystem
  Wendland : Subsystem  mask{NumTerms=NumTerms}
      mask prompts: NumTerms "Number of Polynomial Terms"
  Y : Outport
  J : Outport  Port=2
  wires:
  Constant14/1 -> Wendland/3(Exponent)
  Product4/1 -> Y/1
  Wendland/1(P) -> J/1, Product4/1
  Constant3/1 -> Product4/2
  Math Function4/1 -> Wendland/1(R/S)
  Constant4/1 -> R/2("Centers ")
  X/1 -> R/1(X)
  Constant2/1 -> R/3(S)
  R/1((R/S)^2) -> Math Function4/1
  Constant13/1 -> Wendland/2(PolyTerms)

== system ssc_battery_management_R2020a/Alternator Variants/Alternator_80A_MBC/Alternator/Regulate Voltage/Approximate Derivative/Derivative Gain ==
  In1 : Inport
  Slider Gain : Gain  Gain=gain  SaturateOnIntegerOverflow=on  OutDataTypeStr=Inherit: Same as input  ParamDataTypeStr=Inherit: Same as input
  Out1 : Outport
  wires:
  In1/1 -> Slider Gain/1
  Slider Gain/1 -> Out1/1

== system ssc_battery_management_R2020a/Alternator Variants/Alternator_100A_MBC/Alternator/100A_Max_Current/Constraint Block/Constraints/Constraint ==
  Xin : Inport
  Constraint - conrange : Subsystem  mask(Range Constraint){}
      mask help: This block impements range constraints for MBC models
      mask init:
      | ud = get_param( gcb, 'UserData' );M = ud.M;HW = ud.HW;LB = ud.LB;UB = ud.UB;Scale = ud.Scale;
  switch : Switch  SaturateOnIntegerOverflow=on  InputSameDT=on
  Distance : Outport
  Interior Point : Outport  Port=2
  wires:
  Constraint - conrange/2(Interior Point) -> switch/1
  Constraint - conrange/1(Distance) -> switch/2, Distance/1
  Xin/1 -> Constraint - conrange/1(Xin), switch/3
  switch/1 -> Interior Point/1

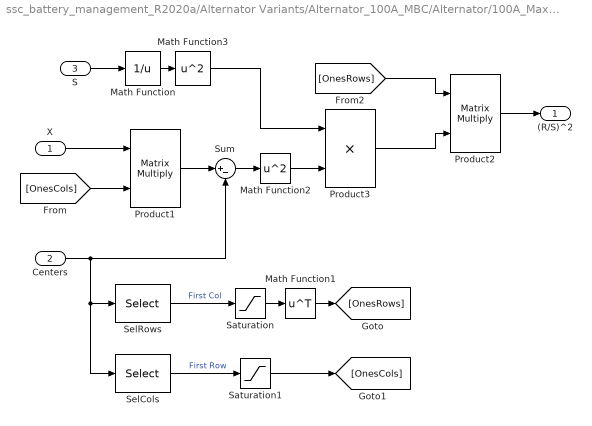
== system ssc_battery_management_R2020a/Alternator Variants/Alternator_100A_MBC/Alternator/100A_Max_Current/xregrbf/rbfwendlandEval/R ==
  X : Inport
  "Centers " : Inport  Port=2
  S : Inport  Port=3
  Math Function : Math  Operator=reciprocal  SignedPower=on  SaturateOnIntegerOverflow=on
  Math Function1 : Math  Operator=transpose  SignedPower=on  SaturateOnIntegerOverflow=on
  Math Function2 : Math  Operator=square  SignedPower=on  SaturateOnIntegerOverflow=on
  Math Function3 : Math  Operator=square  SignedPower=on  SaturateOnIntegerOverflow=on
  Product1 : Product  Multiplication=Matrix(*)  InputSameDT=on  SaturateOnIntegerOverflow=on  OutDataTypeStr=Inherit: Same as first input
  Product2 : Product  Multiplication=Matrix(*)  InputSameDT=on  SaturateOnIntegerOverflow=on  OutDataTypeStr=Inherit: Same as first input
  Product3 : Product  InputSameDT=on  SaturateOnIntegerOverflow=on  OutDataTypeStr=Inherit: Same as first input
  Saturation : Saturate  UpperLimit=1  LowerLimit=1
  Saturation1 : Saturate  UpperLimit=1  LowerLimit=1
  SelCols : Selector  NumberOfDimensions=2  InputPortWidth=3  IndexOptions=Index vector (dialog),Select all  Indices=1,-1  OutputSizes=1
  SelRows : Selector  NumberOfDimensions=2  InputPortWidth=3  IndexOptions=Select all,Index vector (dialog)  Indices=-1,1  OutputSizes=1
  Sum : Sum  Inputs=|+-  InputSameDT=on  SaturateOnIntegerOverflow=on  OutDataTypeStr=Inherit: Same as first input
  (R/S)^2 : Outport
  wires:
  Math Function2/1 -> Product3/2
  Sum/1 -> Math Function2/1
  Product1/1 -> Sum/1
  X/1 -> Product1/1
  [OnesCols] -> Product1/2
  Math Function1/1 -> [OnesRows]
  SelRows/1 -> Saturation/1  "First Col"
  "Centers "/1 -> Sum/2, SelRows/1, SelCols/1
  S/1 -> Math Function/1
  Math Function/1 -> Math Function3/1
  Saturation/1 -> Math Function1/1
  SelCols/1 -> Saturation1/1  "First Row"
  Saturation1/1 -> [OnesCols]
  Math Function3/1 -> Product3/1
  Product3/1 -> Product2/2
  Product2/1 -> (R/S)^2/1
  [OnesRows] -> Product2/1

== system ssc_battery_management_R2020a/Alternator Variants/Alternator_100A_MBC/Alternator/100A_Max_Current/xregrbf/rbfwendlandEval/Wendland ==
  R/S : Inport
  PolyTerms : Inport  Port=2
  Exponent : Inport  Port=3
  Constant : Constant
  Constant1 : Constant  Value=0
  Math Function1 : Math  Operator=pow  SignedPower=on  SaturateOnIntegerOverflow=on
  Product : Product  InputSameDT=on  SaturateOnIntegerOverflow=on  OutDataTypeStr=Inherit: Same as first input
  S-Function : S-Function  FunctionName=WendlandEvalSFnV1  Parameters=NumTerms  SFunctionDeploymentMode=off  EnableBusSupport=off
  Sum : Sum  Inputs=-+|  InputSameDT=on  SaturateOnIntegerOverflow=on  OutDataTypeStr=Inherit: Same as first input
  Switch : Switch  InputSameDT=on
  P : Outport
  wires:
  Product/1 -> P/1
  R/S/1 -> S-Function/2, Sum/1  "R/S"
  PolyTerms/1 -> S-Function/1
  Constant/1 -> Sum/2
  Exponent/1 -> Math Function1/2
  Constant1/1 -> Switch/3
  S-Function/1 -> Product/1
  Sum/1 -> Math Function1/1, Switch/2
  Math Function1/1 -> Switch/1
  Switch/1 -> Product/2

== system ssc_battery_management_R2020a/Alternator Variants/Alternator_100A_MBC/Alternator/100A_Voltage/Constraint Block/Constraints/Constraint ==
  Xin : Inport
  Constraint - conrange : Subsystem  mask(Range Constraint){}
      mask help: This block impements range constraints for MBC models
      mask init:
      | ud = get_param( gcb, 'UserData' );M = ud.M;HW = ud.HW;LB = ud.LB;UB = ud.UB;Scale = ud.Scale;
  switch : Switch  SaturateOnIntegerOverflow=on  InputSameDT=on
  Distance : Outport
  Interior Point : Outport  Port=2
  wires:
  Constraint - conrange/2(Interior Point) -> switch/1
  Constraint - conrange/1(Distance) -> switch/2, Distance/1
  Xin/1 -> Constraint - conrange/1(Xin), switch/3
  switch/1 -> Interior Point/1

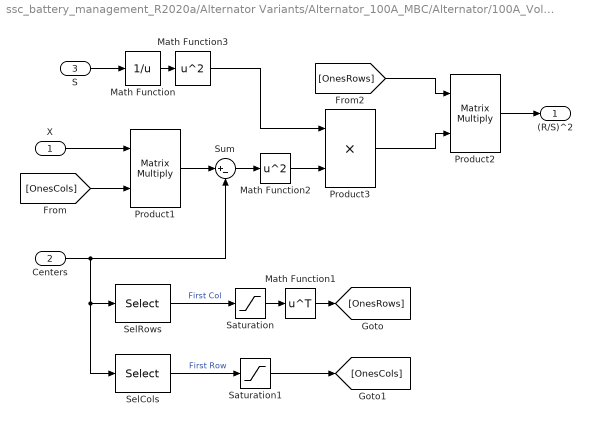
== system ssc_battery_management_R2020a/Alternator Variants/Alternator_100A_MBC/Alternator/100A_Voltage/xregrbf/rbfwendlandEval/R ==
  X : Inport
  "Centers " : Inport  Port=2
  S : Inport  Port=3
  Math Function : Math  Operator=reciprocal  SignedPower=on  SaturateOnIntegerOverflow=on
  Math Function1 : Math  Operator=transpose  SignedPower=on  SaturateOnIntegerOverflow=on
  Math Function2 : Math  Operator=square  SignedPower=on  SaturateOnIntegerOverflow=on
  Math Function3 : Math  Operator=square  SignedPower=on  SaturateOnIntegerOverflow=on
  Product1 : Product  Multiplication=Matrix(*)  InputSameDT=on  SaturateOnIntegerOverflow=on  OutDataTypeStr=Inherit: Same as first input
  Product2 : Product  Multiplication=Matrix(*)  InputSameDT=on  SaturateOnIntegerOverflow=on  OutDataTypeStr=Inherit: Same as first input
  Product3 : Product  InputSameDT=on  SaturateOnIntegerOverflow=on  OutDataTypeStr=Inherit: Same as first input
  Saturation : Saturate  UpperLimit=1  LowerLimit=1
  Saturation1 : Saturate  UpperLimit=1  LowerLimit=1
  SelCols : Selector  NumberOfDimensions=2  InputPortWidth=3  IndexOptions=Index vector (dialog),Select all  Indices=1,-1  OutputSizes=1
  SelRows : Selector  NumberOfDimensions=2  InputPortWidth=3  IndexOptions=Select all,Index vector (dialog)  Indices=-1,1  OutputSizes=1
  Sum : Sum  Inputs=|+-  InputSameDT=on  SaturateOnIntegerOverflow=on  OutDataTypeStr=Inherit: Same as first input
  (R/S)^2 : Outport
  wires:
  Math Function2/1 -> Product3/2
  Sum/1 -> Math Function2/1
  Product1/1 -> Sum/1
  X/1 -> Product1/1
  [OnesCols] -> Product1/2
  Math Function1/1 -> [OnesRows]
  SelRows/1 -> Saturation/1  "First Col"
  "Centers "/1 -> Sum/2, SelRows/1, SelCols/1
  S/1 -> Math Function/1
  Math Function/1 -> Math Function3/1
  Saturation/1 -> Math Function1/1
  SelCols/1 -> Saturation1/1  "First Row"
  Saturation1/1 -> [OnesCols]
  Math Function3/1 -> Product3/1
  Product3/1 -> Product2/2
  Product2/1 -> (R/S)^2/1
  [OnesRows] -> Product2/1
